simulink model "Model_4"  (R2020b)
settings: Solver=VariableStepAuto  StartTime=0.0  StopTime=10.0  RelTol=1e-3
PreLoadFcn:
  | R = 4;
  | L = 2.75E-6;
  | K = 0.0274;
  | J = 3.2284E-6;
  | b = 3.5077E-6;
PostLoadFcn:
  | R = 4;
  | L = 2.75E-6;
  | K = 0.0274;
  | J = 3.2284E-6;
  | b = 3.5077E-6;
settings Model: Creator=samar  LastModifiedBy=Avengers

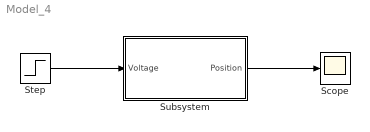
== system Model_4 ==
  Scope : Scope
  Step : Step  SampleTime=0
  Subsystem : Subsystem
  wires:
  Step/1 -> Subsystem/1(Voltage)
  Subsystem/1(Position) -> Scope/1

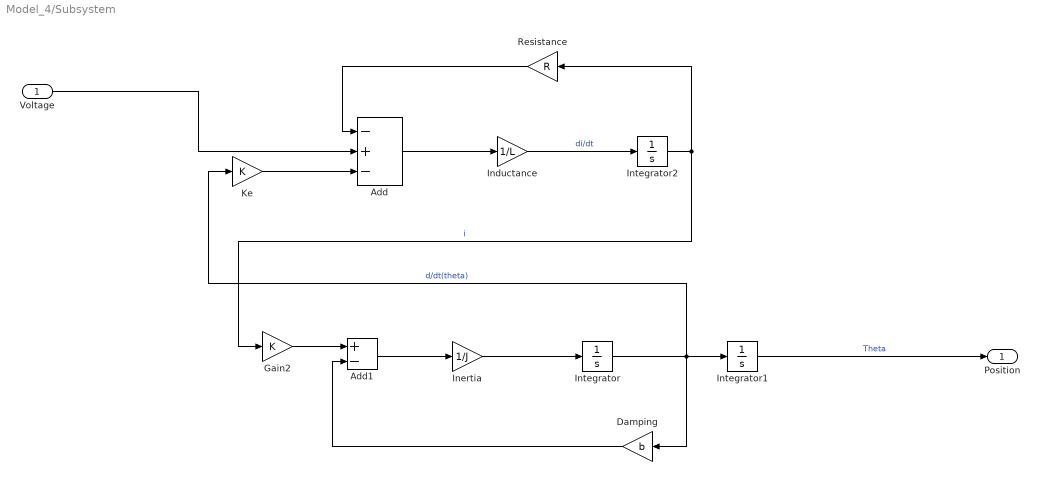
== system Model_4/Subsystem ==
  Voltage : Inport
  Add : Sum  Inputs=-+-
  Add1 : Sum  Inputs=+-
  Damping : Gain  Gain=b
  Gain2 : Gain  Gain=K
  Inductance : Gain  Gain=1/L
  Inertia : Gain  Gain=1/J
  Integrator : Integrator
  Integrator1 : Integrator
  Integrator2 : Integrator
  Ke : Gain  Gain=K
  Resistance : Gain  Gain=R
  Position : Outport
  wires:
  Integrator/1 -> Ke/1, Integrator1/1, Damping/1  "d/dt(theta)"
  Damping/1 -> Add1/2
  Voltage/1 -> Add/2
  Integrator1/1 -> Position/1  "Theta"
  Add/1 -> Inductance/1
  Ke/1 -> Add/3
  Add1/1 -> Inertia/1
  Gain2/1 -> Add1/1
  Integrator2/1 -> Gain2/1, Resistance/1  "i"
  Resistance/1 -> Add/1
  Inductance/1 -> Integrator2/1  "di/dt"
  Inertia/1 -> Integrator/1
